simulink library "xpclib"  (Simulink 6.0)
settings: Solver=ode45  SolverMode=SingleTasking  StartTime=0.0  StopTime=10.0  RelTol=1e-3
values from neighbouring files (symbols this model uses):
  base = get_param( gcb, 'base' )    [maddiamondmm.m]    (also in maddiamondmm32.m; maddiamondmm32frame.m; maddsmm16at.m; malaim16.m = hex2dec(baseaddress(3:end)))
  data = ''    [mbwaudpmc.m]
  irq = params{3}    [mbaseserialmask.m]
  port = [0,1]    [canfifofilterutil.m]    (also in mbaseserialmask.m = str2num(get_param( gcb, 'port' )))
undefined symbols (not defined in the file or in its folder): CIO, devid, DIO24, genixlib, get, handlers, mbaseserialmask, mbwaudpmc, mdacbpcidas, mdiamondemeraldmask, mgenix, mmodemcontrol, mquamask, mrs232, msc150checks, mtargetboxleds, mtargetboxwatchdog, mxpccan, PCI, sizeof, vendid
libraries: xpclib x384, simulink x6
(part 7 of 7)

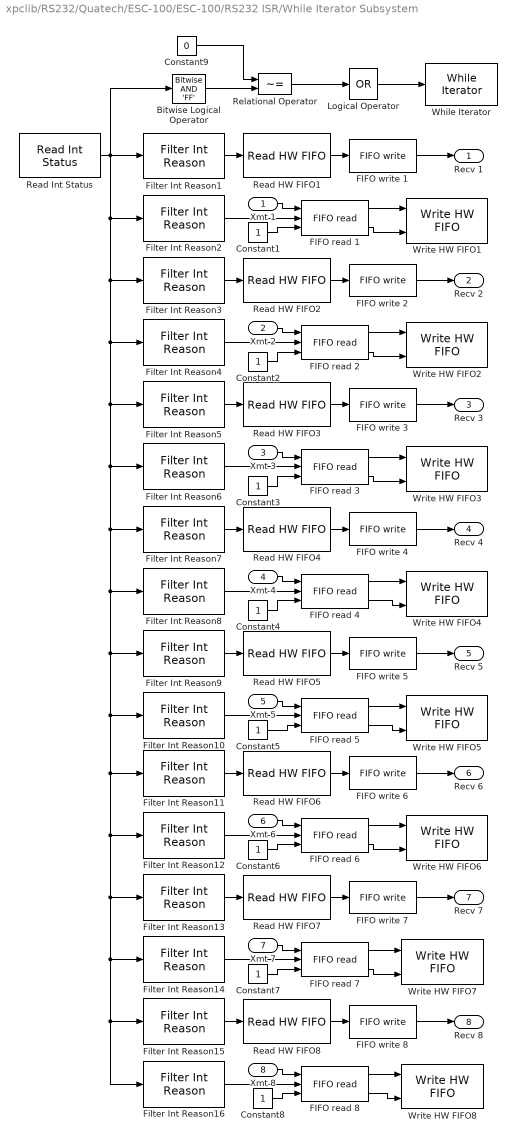
== system xpclib/RS232/Quatech/ESC-100/ESC-100/RS232 ISR/While Iterator Subsystem ==
  Xmt 1 : Inport  LatchInput=off
  Xmt 2 : Inport  Port=2  LatchInput=off
  Xmt 3 : Inport  Port=3  LatchInput=off
  Xmt 4 : Inport  Port=4  LatchInput=off
  Xmt 5 : Inport  Port=5  LatchInput=off
  Xmt 6 : Inport  Port=6  LatchInput=off
  Xmt 7 : Inport  Port=7  LatchInput=off
  Xmt 8 : Inport  Port=8  LatchInput=off
  Bitwise Logical Operator : simulink/Logic and Bit Operations/Bitwise Operator  logicop=AND  UseBitMask=on  BitMask='FF'  BitMaskRealWorld=Stored Integer
  Constant{1..8} (8 alike) : Constant  OutDataTypeMode=uint32
  Constant9 : Constant  Value=0  OutDataTypeMode=uint32
  FIFO read {1..8} (8 alike) : xpclib/RS232/FIFO read   maxsize=60  minsize=1  usedelimiter=off  delimiter=13  outputtype=count+32 bit uint  enable=on  enableout=on  sampletime=-1
  FIFO write 1 : xpclib/RS232/FIFO write   size=1024  inputtype=count+32 bit uint  present=off  sampletime=-1  id=RCV channel 1, IRQ 7
  FIFO write 2 : xpclib/RS232/FIFO write   size=1024  inputtype=count+32 bit uint  present=off  sampletime=-1  id=RCV channel 2, IRQ 7
  FIFO write 3 : xpclib/RS232/FIFO write   size=1024  inputtype=count+32 bit uint  present=off  sampletime=-1  id=RCV channel 3, IRQ 7
  FIFO write 4 : xpclib/RS232/FIFO write   size=1024  inputtype=count+32 bit uint  present=off  sampletime=-1  id=RCV channel 4, IRQ 7
  FIFO write 5 : xpclib/RS232/FIFO write   size=1024  inputtype=count+32 bit uint  present=off  sampletime=-1  id=RCV channel 5, IRQ 7
  FIFO write 6 : xpclib/RS232/FIFO write   size=1024  inputtype=count+32 bit uint  present=off  sampletime=-1  id=RCV channel 6, IRQ 7
  FIFO write 7 : xpclib/RS232/FIFO write   size=1024  inputtype=count+32 bit uint  present=off  sampletime=-1  id=RCV channel 7, IRQ 7
  FIFO write 8 : xpclib/RS232/FIFO write   size=1024  inputtype=count+32 bit uint  present=off  sampletime=-1  id=RCV channel 8, IRQ 7
  Filter Int Reason1 : xpclib/RS232/Quatech/ESC-100/ESC-100 Internal blocks/Filter Int Reason  port=1  value=Receive data
  Filter Int Reason10 : xpclib/RS232/Quatech/ESC-100/ESC-100 Internal blocks/Filter Int Reason  port=5  value=Transmitter empty
  Filter Int Reason11 : xpclib/RS232/Quatech/ESC-100/ESC-100 Internal blocks/Filter Int Reason  port=6  value=Receive data
  Filter Int Reason12 : xpclib/RS232/Quatech/ESC-100/ESC-100 Internal blocks/Filter Int Reason  port=6  value=Transmitter empty
  Filter Int Reason13 : xpclib/RS232/Quatech/ESC-100/ESC-100 Internal blocks/Filter Int Reason  port=7  value=Receive data
  Filter Int Reason14 : xpclib/RS232/Quatech/ESC-100/ESC-100 Internal blocks/Filter Int Reason  port=7  value=Transmitter empty
  Filter Int Reason15 : xpclib/RS232/Quatech/ESC-100/ESC-100 Internal blocks/Filter Int Reason  port=8  value=Receive data
  Filter Int Reason16 : xpclib/RS232/Quatech/ESC-100/ESC-100 Internal blocks/Filter Int Reason  port=8  value=Transmitter empty
  Filter Int Reason2 : xpclib/RS232/Quatech/ESC-100/ESC-100 Internal blocks/Filter Int Reason  port=1  value=Transmitter empty
  Filter Int Reason3 : xpclib/RS232/Quatech/ESC-100/ESC-100 Internal blocks/Filter Int Reason  port=2  value=Receive data
  Filter Int Reason4 : xpclib/RS232/Quatech/ESC-100/ESC-100 Internal blocks/Filter Int Reason  port=2  value=Transmitter empty
  Filter Int Reason5 : xpclib/RS232/Quatech/ESC-100/ESC-100 Internal blocks/Filter Int Reason  port=3  value=Receive data
  Filter Int Reason6 : xpclib/RS232/Quatech/ESC-100/ESC-100 Internal blocks/Filter Int Reason  port=3  value=Transmitter empty
  Filter Int Reason7 : xpclib/RS232/Quatech/ESC-100/ESC-100 Internal blocks/Filter Int Reason  port=4  value=Receive data
  Filter Int Reason8 : xpclib/RS232/Quatech/ESC-100/ESC-100 Internal blocks/Filter Int Reason  port=4  value=Transmitter empty
  Filter Int Reason9 : xpclib/RS232/Quatech/ESC-100/ESC-100 Internal blocks/Filter Int Reason  port=5  value=Receive data
  Logical Operator : Logic  Operator=OR  Inputs=1  AllPortsSameDT=off
  Read HW FIFO1 : xpclib/RS232/Quatech/ESC-100/ESC-100 Internal blocks/Read HW FIFO  port=1  flush=on  slot=subslot
  Read HW FIFO2 : xpclib/RS232/Quatech/ESC-100/ESC-100 Internal blocks/Read HW FIFO  port=2  flush=on  slot=subslot
  Read HW FIFO3 : xpclib/RS232/Quatech/ESC-100/ESC-100 Internal blocks/Read HW FIFO  port=3  flush=on  slot=subslot
  Read HW FIFO4 : xpclib/RS232/Quatech/ESC-100/ESC-100 Internal blocks/Read HW FIFO  port=4  flush=on  slot=subslot
  Read HW FIFO5 : xpclib/RS232/Quatech/ESC-100/ESC-100 Internal blocks/Read HW FIFO  port=5  flush=on  slot=subslot
  Read HW FIFO6 : xpclib/RS232/Quatech/ESC-100/ESC-100 Internal blocks/Read HW FIFO  port=6  flush=on  slot=subslot
  Read HW FIFO7 : xpclib/RS232/Quatech/ESC-100/ESC-100 Internal blocks/Read HW FIFO  port=7  flush=on  slot=subslot
  Read HW FIFO8 : xpclib/RS232/Quatech/ESC-100/ESC-100 Internal blocks/Read HW FIFO  port=8  flush=on  slot=subslot
  Read Int Status : xpclib/RS232/Quatech/ESC-100/ESC-100 Internal blocks/Read Int Status  slot=subslot
  Relational Operator : RelationalOperator  Operator=~=
  While Iterator : WhileIterator  MaxIters=65  WhileBlockType=do-while
  Write HW FIFO1 : xpclib/RS232/Quatech/ESC-100/ESC-100 Internal blocks/Write HW FIFO  port=1  slot=subslot
  Write HW FIFO2 : xpclib/RS232/Quatech/ESC-100/ESC-100 Internal blocks/Write HW FIFO  port=2  slot=subslot
  Write HW FIFO3 : xpclib/RS232/Quatech/ESC-100/ESC-100 Internal blocks/Write HW FIFO  port=3  slot=subslot
  Write HW FIFO4 : xpclib/RS232/Quatech/ESC-100/ESC-100 Internal blocks/Write HW FIFO  port=4  slot=subslot
  Write HW FIFO5 : xpclib/RS232/Quatech/ESC-100/ESC-100 Internal blocks/Write HW FIFO  port=5  slot=subslot
  Write HW FIFO6 : xpclib/RS232/Quatech/ESC-100/ESC-100 Internal blocks/Write HW FIFO  port=6  slot=subslot
  Write HW FIFO7 : xpclib/RS232/Quatech/ESC-100/ESC-100 Internal blocks/Write HW FIFO  port=7  slot=subslot
  Write HW FIFO8 : xpclib/RS232/Quatech/ESC-100/ESC-100 Internal blocks/Write HW FIFO  port=8  slot=subslot
  Recv 1 : Outport
  Recv 2 : Outport  Port=2
  Recv 3 : Outport  Port=3
  Recv 4 : Outport  Port=4
  Recv 5 : Outport  Port=5
  Recv 6 : Outport  Port=6
  Recv 7 : Outport  Port=7
  Recv 8 : Outport  Port=8
  wires:
  Read Int Status/1 -> Filter Int Reason1/1, Filter Int Reason2/1, Filter Int Reason3/1, Filter Int Reason4/1, Filter Int Reason5/1, Filter Int Reason6/1, Filter Int Reason7/1, Filter Int Reason8/1, Filter Int Reason9/1, Filter Int Reason10/1, Filter Int Reason11/1, Filter Int Reason12/1, Filter Int Reason13/1, Filter Int Reason14/1, Filter Int Reason16/1, Filter Int Reason15/1, Bitwise Logical Operator/1
  Filter Int Reason1/1 -> Read HW FIFO1/1
  FIFO write 1/1 -> Recv 1/1
  Read HW FIFO1/1 -> FIFO write 1/1
  Filter Int Reason2/1 -> FIFO read 1/2
  Xmt 1/1 -> FIFO read 1/1
  Filter Int Reason3/1 -> Read HW FIFO2/1
  FIFO write 2/1 -> Recv 2/1
  Read HW FIFO2/1 -> FIFO write 2/1
  Filter Int Reason4/1 -> FIFO read 2/2
  Xmt 2/1 -> FIFO read 2/1
  Filter Int Reason5/1 -> Read HW FIFO3/1
  FIFO write 3/1 -> Recv 3/1
  Read HW FIFO3/1 -> FIFO write 3/1
  Filter Int Reason6/1 -> FIFO read 3/2
  Xmt 3/1 -> FIFO read 3/1
  Filter Int Reason7/1 -> Read HW FIFO4/1
  FIFO write 4/1 -> Recv 4/1
  Read HW FIFO4/1 -> FIFO write 4/1
  Filter Int Reason8/1 -> FIFO read 4/2
  Xmt 4/1 -> FIFO read 4/1
  Filter Int Reason9/1 -> Read HW FIFO5/1
  FIFO write 5/1 -> Recv 5/1
  Read HW FIFO5/1 -> FIFO write 5/1
  Filter Int Reason10/1 -> FIFO read 5/2
  Xmt 5/1 -> FIFO read 5/1
  Filter Int Reason11/1 -> Read HW FIFO6/1
  FIFO write 6/1 -> Recv 6/1
  Read HW FIFO6/1 -> FIFO write 6/1
  Filter Int Reason12/1 -> FIFO read 6/2
  Xmt 6/1 -> FIFO read 6/1
  Filter Int Reason13/1 -> Read HW FIFO7/1
  FIFO write 7/1 -> Recv 7/1
  Read HW FIFO7/1 -> FIFO write 7/1
  Filter Int Reason14/1 -> FIFO read 7/2
  Xmt 7/1 -> FIFO read 7/1
  Filter Int Reason15/1 -> Read HW FIFO8/1
  FIFO write 8/1 -> Recv 8/1
  Read HW FIFO8/1 -> FIFO write 8/1
  Filter Int Reason16/1 -> FIFO read 8/2
  Xmt 8/1 -> FIFO read 8/1
  FIFO read 8/1 -> Write HW FIFO8/1
  FIFO read 8/2 -> Write HW FIFO8/2
  FIFO read 7/1 -> Write HW FIFO7/1
  FIFO read 7/2 -> Write HW FIFO7/2
  FIFO read 6/1 -> Write HW FIFO6/1
  FIFO read 6/2 -> Write HW FIFO6/2
  FIFO read 5/1 -> Write HW FIFO5/1
  FIFO read 5/2 -> Write HW FIFO5/2
  FIFO read 4/1 -> Write HW FIFO4/1
  FIFO read 4/2 -> Write HW FIFO4/2
  FIFO read 3/1 -> Write HW FIFO3/1
  FIFO read 3/2 -> Write HW FIFO3/2
  FIFO read 2/1 -> Write HW FIFO2/1
  FIFO read 2/2 -> Write HW FIFO2/2
  FIFO read 1/1 -> Write HW FIFO1/1
  FIFO read 1/2 -> Write HW FIFO1/2
  Constant1/1 -> FIFO read 1/3
  Constant2/1 -> FIFO read 2/3
  Constant3/1 -> FIFO read 3/3
  Constant4/1 -> FIFO read 4/3
  Constant5/1 -> FIFO read 5/3
  Constant6/1 -> FIFO read 6/3
  Constant7/1 -> FIFO read 7/3
  Constant8/1 -> FIFO read 8/3
  Logical Operator/1 -> While Iterator/1
  Relational Operator/1 -> Logical Operator/1
  Bitwise Logical Operator/1 -> Relational Operator/2
  Constant9/1 -> Relational Operator/1

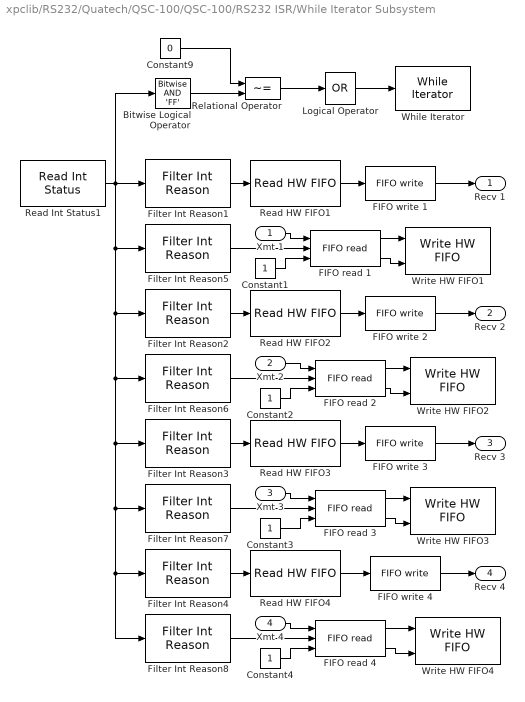
== system xpclib/RS232/Quatech/QSC-100/QSC-100/RS232 ISR/While Iterator Subsystem ==
  Xmt 1 : Inport  LatchInput=off
  Xmt 2 : Inport  Port=2  LatchInput=off
  Xmt 3 : Inport  Port=3  LatchInput=off
  Xmt 4 : Inport  Port=4  LatchInput=off
  Bitwise Logical Operator : simulink/Logic and Bit Operations/Bitwise Operator  logicop=AND  UseBitMask=on  BitMask='FF'  BitMaskRealWorld=Stored Integer
  Constant{1..4} (4 alike) : Constant  OutDataTypeMode=uint32
  Constant9 : Constant  Value=0  OutDataTypeMode=uint32
  FIFO read {1..4} (4 alike) : xpclib/RS232/FIFO read   maxsize=60  minsize=1  usedelimiter=off  delimiter=13  outputtype=count+32 bit uint  enable=on  enableout=on  sampletime=-1
  FIFO write 1 : xpclib/RS232/FIFO write   size=1024  inputtype=count+32 bit uint  present=off  sampletime=-1  id=RCV channel 1, IRQ 7
  FIFO write 2 : xpclib/RS232/FIFO write   size=1024  inputtype=count+32 bit uint  present=off  sampletime=-1  id=RCV channel 2, IRQ 7
  FIFO write 3 : xpclib/RS232/FIFO write   size=1024  inputtype=count+32 bit uint  present=off  sampletime=-1  id=RCV channel 3, IRQ 7
  FIFO write 4 : xpclib/RS232/FIFO write   size=1024  inputtype=count+32 bit uint  present=off  sampletime=-1  id=RCV channel 4, IRQ 7
  Filter Int Reason1 : xpclib/RS232/Quatech/QSC-100/QSC-100 Internal  blocks/Filter Int Reason  port=1  value=Receive data
  Filter Int Reason2 : xpclib/RS232/Quatech/QSC-100/QSC-100 Internal  blocks/Filter Int Reason  port=2  value=Receive data
  Filter Int Reason3 : xpclib/RS232/Quatech/QSC-100/QSC-100 Internal  blocks/Filter Int Reason  port=3  value=Receive data
  Filter Int Reason4 : xpclib/RS232/Quatech/QSC-100/QSC-100 Internal  blocks/Filter Int Reason  port=4  value=Receive data
  Filter Int Reason5 : xpclib/RS232/Quatech/QSC-100/QSC-100 Internal  blocks/Filter Int Reason  port=1  value=Transmitter empty
  Filter Int Reason6 : xpclib/RS232/Quatech/QSC-100/QSC-100 Internal  blocks/Filter Int Reason  port=2  value=Transmitter empty
  Filter Int Reason7 : xpclib/RS232/Quatech/QSC-100/QSC-100 Internal  blocks/Filter Int Reason  port=3  value=Transmitter empty
  Filter Int Reason8 : xpclib/RS232/Quatech/QSC-100/QSC-100 Internal  blocks/Filter Int Reason  port=4  value=Transmitter empty
  Logical Operator : Logic  Operator=OR  Inputs=1  AllPortsSameDT=off
  Read HW FIFO1 : xpclib/RS232/Quatech/QSC-100/QSC-100 Internal  blocks/Read HW FIFO  port=1  flush=on  slot=subslot
  Read HW FIFO2 : xpclib/RS232/Quatech/QSC-100/QSC-100 Internal  blocks/Read HW FIFO  port=2  flush=on  slot=subslot
  Read HW FIFO3 : xpclib/RS232/Quatech/QSC-100/QSC-100 Internal  blocks/Read HW FIFO  port=3  flush=on  slot=subslot
  Read HW FIFO4 : xpclib/RS232/Quatech/QSC-100/QSC-100 Internal  blocks/Read HW FIFO  port=4  flush=on  slot=subslot
  Read Int Status1 : xpclib/RS232/Quatech/QSC-100/QSC-100 Internal  blocks/Read Int Status  slot=subslot
  Relational Operator : RelationalOperator  Operator=~=
  While Iterator : WhileIterator  MaxIters=65  WhileBlockType=do-while
  Write HW FIFO1 : xpclib/RS232/Quatech/QSC-100/QSC-100 Internal  blocks/Write HW FIFO  port=1  slot=subslot
  Write HW FIFO2 : xpclib/RS232/Quatech/QSC-100/QSC-100 Internal  blocks/Write HW FIFO  port=2  slot=subslot
  Write HW FIFO3 : xpclib/RS232/Quatech/QSC-100/QSC-100 Internal  blocks/Write HW FIFO  port=3  slot=subslot
  Write HW FIFO4 : xpclib/RS232/Quatech/QSC-100/QSC-100 Internal  blocks/Write HW FIFO  port=4  slot=subslot
  Recv 1 : Outport
  Recv 2 : Outport  Port=2
  Recv 3 : Outport  Port=3
  Recv 4 : Outport  Port=4
  wires:
  Xmt 4/1 -> FIFO read 4/1
  Filter Int Reason8/1 -> FIFO read 4/2
  Read HW FIFO4/1 -> FIFO write 4/1
  FIFO write 4/1 -> Recv 4/1
  Filter Int Reason4/1 -> Read HW FIFO4/1
  Xmt 3/1 -> FIFO read 3/1
  Filter Int Reason7/1 -> FIFO read 3/2
  Read HW FIFO3/1 -> FIFO write 3/1
  FIFO write 3/1 -> Recv 3/1
  Filter Int Reason3/1 -> Read HW FIFO3/1
  Xmt 2/1 -> FIFO read 2/1
  Filter Int Reason6/1 -> FIFO read 2/2
  Read HW FIFO2/1 -> FIFO write 2/1
  FIFO write 2/1 -> Recv 2/1
  Filter Int Reason2/1 -> Read HW FIFO2/1
  Xmt 1/1 -> FIFO read 1/1
  Filter Int Reason5/1 -> FIFO read 1/2
  Read HW FIFO1/1 -> FIFO write 1/1
  FIFO write 1/1 -> Recv 1/1
  Filter Int Reason1/1 -> Read HW FIFO1/1
  Read Int Status1/1 -> Filter Int Reason1/1, Filter Int Reason5/1, Filter Int Reason2/1, Filter Int Reason6/1, Filter Int Reason3/1, Filter Int Reason7/1, Filter Int Reason8/1, Filter Int Reason4/1, Bitwise Logical Operator/1
  FIFO read 4/1 -> Write HW FIFO4/1
  FIFO read 4/2 -> Write HW FIFO4/2
  FIFO read 3/1 -> Write HW FIFO3/1
  FIFO read 3/2 -> Write HW FIFO3/2
  FIFO read 2/1 -> Write HW FIFO2/1
  FIFO read 2/2 -> Write HW FIFO2/2
  FIFO read 1/1 -> Write HW FIFO1/1
  FIFO read 1/2 -> Write HW FIFO1/2
  Constant1/1 -> FIFO read 1/3
  Constant2/1 -> FIFO read 2/3
  Constant3/1 -> FIFO read 3/3
  Constant4/1 -> FIFO read 4/3
  Logical Operator/1 -> While Iterator/1
  Relational Operator/1 -> Logical Operator/1
  Bitwise Logical Operator/1 -> Relational Operator/2
  Constant9/1 -> Relational Operator/1

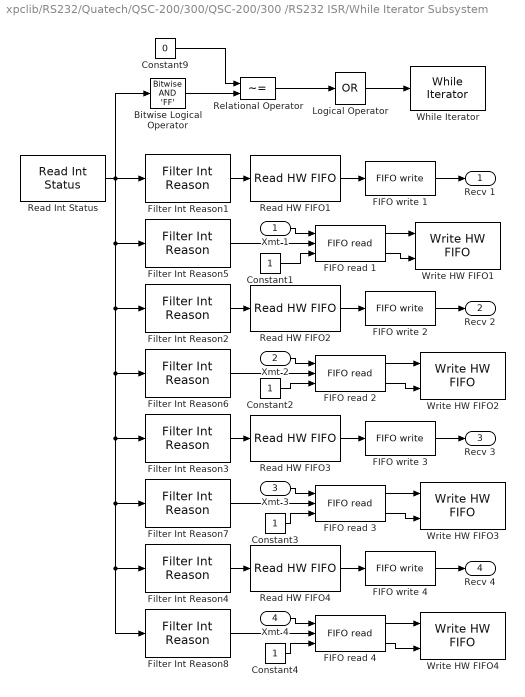
== system xpclib/RS232/Quatech/QSC-200/300/QSC-200/300 /RS232 ISR/While Iterator Subsystem ==
  Xmt 1 : Inport  LatchInput=off
  Xmt 2 : Inport  Port=2  LatchInput=off
  Xmt 3 : Inport  Port=3  LatchInput=off
  Xmt 4 : Inport  Port=4  LatchInput=off
  Bitwise Logical Operator : simulink/Logic and Bit Operations/Bitwise Operator  logicop=AND  UseBitMask=on  BitMask='FF'  BitMaskRealWorld=Stored Integer
  Constant{1..4} (4 alike) : Constant  OutDataTypeMode=uint32
  Constant9 : Constant  Value=0  OutDataTypeMode=uint32
  FIFO read {1..4} (4 alike) : xpclib/RS232/FIFO read   maxsize=60  minsize=1  usedelimiter=off  delimiter=13  outputtype=count+32 bit uint  enable=on  enableout=on  sampletime=-1
  FIFO write {1..4} (4 alike) : xpclib/RS232/FIFO write   size=1024  inputtype=count+32 bit uint  present=off  sampletime=-1
  Filter Int Reason1 : xpclib/RS232/Quatech/QSC-200//300/QSC-200//300 Internal  blocks1/Filter Int Reason  port=1  value=Receive data
  Filter Int Reason2 : xpclib/RS232/Quatech/QSC-200//300/QSC-200//300 Internal  blocks1/Filter Int Reason  port=2  value=Receive data
  Filter Int Reason3 : xpclib/RS232/Quatech/QSC-200//300/QSC-200//300 Internal  blocks1/Filter Int Reason  port=3  value=Receive data
  Filter Int Reason4 : xpclib/RS232/Quatech/QSC-200//300/QSC-200//300 Internal  blocks1/Filter Int Reason  port=4  value=Receive data
  Filter Int Reason5 : xpclib/RS232/Quatech/QSC-200//300/QSC-200//300 Internal  blocks1/Filter Int Reason  port=1  value=Transmitter empty
  Filter Int Reason6 : xpclib/RS232/Quatech/QSC-200//300/QSC-200//300 Internal  blocks1/Filter Int Reason  port=2  value=Transmitter empty
  Filter Int Reason7 : xpclib/RS232/Quatech/QSC-200//300/QSC-200//300 Internal  blocks1/Filter Int Reason  port=3  value=Transmitter empty
  Filter Int Reason8 : xpclib/RS232/Quatech/QSC-200//300/QSC-200//300 Internal  blocks1/Filter Int Reason  port=4  value=Transmitter empty
  Logical Operator : Logic  Operator=OR  Inputs=1  AllPortsSameDT=off
  Read HW FIFO1 : xpclib/RS232/Quatech/QSC-200//300/QSC-200//300 Internal  blocks1/Read HW FIFO  port=1  flush=on  slot=subslot
  Read HW FIFO2 : xpclib/RS232/Quatech/QSC-200//300/QSC-200//300 Internal  blocks1/Read HW FIFO  port=2  flush=on  slot=subslot
  Read HW FIFO3 : xpclib/RS232/Quatech/QSC-200//300/QSC-200//300 Internal  blocks1/Read HW FIFO  port=3  flush=on  slot=subslot
  Read HW FIFO4 : xpclib/RS232/Quatech/QSC-200//300/QSC-200//300 Internal  blocks1/Read HW FIFO  port=4  flush=on  slot=subslot
  Read Int Status : xpclib/RS232/Quatech/QSC-200//300/QSC-200//300 Internal  blocks1/Read Int Status  slot=subslot
  Relational Operator : RelationalOperator  Operator=~=
  While Iterator : WhileIterator  MaxIters=65  WhileBlockType=do-while
  Write HW FIFO1 : xpclib/RS232/Quatech/QSC-200//300/QSC-200//300 Internal  blocks1/Write HW FIFO  port=1  onxmt=None  slot=subslot
  Write HW FIFO2 : xpclib/RS232/Quatech/QSC-200//300/QSC-200//300 Internal  blocks1/Write HW FIFO  port=2  onxmt=None  slot=subslot
  Write HW FIFO3 : xpclib/RS232/Quatech/QSC-200//300/QSC-200//300 Internal  blocks1/Write HW FIFO  port=3  onxmt=None  slot=subslot
  Write HW FIFO4 : xpclib/RS232/Quatech/QSC-200//300/QSC-200//300 Internal  blocks1/Write HW FIFO  port=4  onxmt=None  slot=subslot
  Recv 1 : Outport
  Recv 2 : Outport  Port=2
  Recv 3 : Outport  Port=3
  Recv 4 : Outport  Port=4
  wires:
  Read Int Status/1 -> Filter Int Reason1/1, Filter Int Reason5/1, Filter Int Reason2/1, Filter Int Reason6/1, Filter Int Reason3/1, Filter Int Reason7/1, Filter Int Reason8/1, Filter Int Reason4/1, Bitwise Logical Operator/1
  Filter Int Reason1/1 -> Read HW FIFO1/1
  FIFO write 1/1 -> Recv 1/1
  Read HW FIFO1/1 -> FIFO write 1/1
  Filter Int Reason5/1 -> FIFO read 1/2
  Xmt 1/1 -> FIFO read 1/1
  Filter Int Reason2/1 -> Read HW FIFO2/1
  FIFO write 2/1 -> Recv 2/1
  Read HW FIFO2/1 -> FIFO write 2/1
  Filter Int Reason6/1 -> FIFO read 2/2
  Xmt 2/1 -> FIFO read 2/1
  Filter Int Reason3/1 -> Read HW FIFO3/1
  FIFO write 3/1 -> Recv 3/1
  Read HW FIFO3/1 -> FIFO write 3/1
  Filter Int Reason7/1 -> FIFO read 3/2
  Xmt 3/1 -> FIFO read 3/1
  Filter Int Reason4/1 -> Read HW FIFO4/1
  FIFO write 4/1 -> Recv 4/1
  Read HW FIFO4/1 -> FIFO write 4/1
  Filter Int Reason8/1 -> FIFO read 4/2
  Xmt 4/1 -> FIFO read 4/1
  FIFO read 4/1 -> Write HW FIFO4/1
  FIFO read 3/1 -> Write HW FIFO3/1
  FIFO read 3/2 -> Write HW FIFO3/2
  FIFO read 2/1 -> Write HW FIFO2/1
  FIFO read 1/1 -> Write HW FIFO1/1
  FIFO read 1/2 -> Write HW FIFO1/2
  FIFO read 2/2 -> Write HW FIFO2/2
  FIFO read 4/2 -> Write HW FIFO4/2
  Constant1/1 -> FIFO read 1/3
  Constant2/1 -> FIFO read 2/3
  Constant3/1 -> FIFO read 3/3
  Constant4/1 -> FIFO read 4/3
  Logical Operator/1 -> While Iterator/1
  Relational Operator/1 -> Logical Operator/1
  Bitwise Logical Operator/1 -> Relational Operator/2
  Constant9/1 -> Relational Operator/1
